simulink model "NormalChopper"  (R2018a)
settings: Solver=VariableStepAuto  StartTime=0.0  StopTime=0.6  RelTol=1e-3  AbsTol=1e-3  EnableMultiTasking=on
values from neighbouring files (symbols this model uses):
  C1 = 200e-6    (= 0.0002)    [test_TFCheck.m]
  C1_ESL = 1e-9    (= 1e-09)    [test_TFCheck.m]
  C1_ESR = 1e-3    (= 0.001)    [test_TFCheck.m]
  C2 = 1000e-6    (= 0.001)    [test_TFCheck.m]
  C2_ESL = 1e-9    (= 1e-09)    [test_TFCheck.m]
  C2_ESR = 1e-3    (= 0.001)    [test_TFCheck.m]
  C_smooth = 400e-6    (= 0.0004)    [test_TFCheck.m]
  current_source = 5.0    (= 5)    [test_TFCheck.m]
  L1 = 1e-6    (= 1e-06)    [test_TFCheck.m]
  L1_R = 1e-3    (= 0.001)    [test_TFCheck.m]
  L2 = 1e-6    (= 1e-06)    [test_TFCheck.m]
  L2_R = 1e-3    (= 0.001)    [test_TFCheck.m]
  L_cable = 10e-6    (= 1e-05)    [test_TFCheck.m]
  L_reactor = 200e-6    (= 0.0002)    [test_TFCheck.m]
  R_cable = 12e-3    (= 0.012)    [test_TFCheck.m]
  R_reactor = 30e-3    (= 0.03)    [test_TFCheck.m]
  sample_time = 1e-6    (= 1e-06)    [test_TFCheck.m]
  SW_duty = 0.5    [ChopperRmsSIm.m]    (also in test_TFCheck.m)
  Vdc = 50    [test_TFCheck.m]
libraries: powerlib x22, powerlib_meascontrol x1
settings Model: Creator=snow_  LastModifiedBy=snow_
settings SolverCC: AutoScaleAbsTol=off
settings DataIOCC: LimitDataPoints=on  MaxDataPoints=10000
settings OptimizationCC: LifeSpan=inf
settings DebuggingCC: AllowSymbolicDim=off  SFUnexpectedBacktrackingDiag=warning  SFNoUnconditionalDefaultTransitionDiag=warning  SFExecutionAtInitializationDiag=none
settings CodeAppCC: StateflowObjectComments=on
settings GRTTargetCC: TargetLangStandard=C89/C90 (ANSI)  GeneratePreprocessorConditionals=Disable all
settings ConfigComp: CovMetricSettings=dw  CovHtmlReporting=on  CovSaveCumulativeToWorkspaceVar=on  CovSaveSingleToWorkspaceVar=on  CovExternalEMLEnable=off  CovSFcnEnable=off
settings SimscapeCC: SimscapeLogType=all  SimscapeLogDataHistory=10000

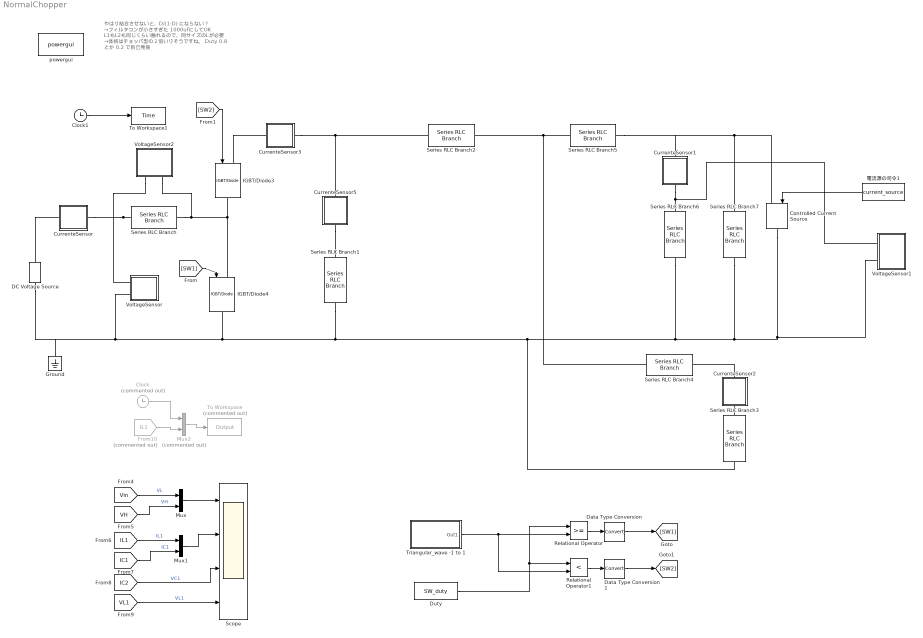
== system NormalChopper ==
  note: やはり結合させないと、D/(1-D)　にならない？
      | →フィルタコンが小さすぎた　1000uFにしてOK
      |
      | L1もL2も同じくらい触れるので、同サイズのLが必要
      | →体格はチョッパ型の２倍いりそうですね。
      |
      | Duty 0.8 とか　0.2 で自己発振
  Clock : Clock  Commented=on
  Clock1 : Clock
  Controlled Current Source : powerlib/Electrical Sources/Controlled Current Source  Initialize=on  Source_Type=AC  Amplitude=0  Phase=0  Frequency=0  Measurements=None
  CurrenteSensor : Subsystem  mask{VariableName=IL1, SampleTime=sample_time}
      mask prompts: VariableName "Simulink:blkprm_prompts:ToWksVarName"
      settings: AttributesFormatString=%<VariableName>
      mask TypeOptions VariableName: To Workspace1/VariableName | Goto/GotoTag
      mask DialogControl VariableName Prompt: 変数名:
      mask Display:
      | disp("Current \n Sensor")
      | port_label('lconn', 1, '+')
      | port_label('rconn', 1, '-')
      | 
      | 
      | %set_param([gcb '/Goto'],'GotoTag',VariableName) % これは使えないっぽい
  CurrenteSensor1 : Subsystem  mask{VariableName=IC2, SampleTime=sample_time}
      mask prompts: VariableName "Simulink:blkprm_prompts:ToWksVarName"
      settings: AttributesFormatString=%<VariableName>
      mask TypeOptions VariableName: To Workspace1/VariableName | Goto/GotoTag
      mask DialogControl VariableName Prompt: 変数名:
      mask Display:
      | disp("Current \n Sensor")
      | port_label('lconn', 1, '+')
      | port_label('rconn', 1, '-')
      | 
      | 
      | %set_param([gcb '/Goto'],'GotoTag',VariableName) % これは使えないっぽい
  CurrenteSensor2 : Subsystem  mask{VariableName=IC3, SampleTime=sample_time}
      mask prompts: VariableName "Simulink:blkprm_prompts:ToWksVarName"
      settings: AttributesFormatString=%<VariableName>
      mask TypeOptions VariableName: To Workspace1/VariableName | Goto/GotoTag
      mask DialogControl VariableName Prompt: 変数名:
      mask Display:
      | disp("Current \n Sensor")
      | port_label('lconn', 1, '+')
      | port_label('rconn', 1, '-')
      | 
      | 
      | %set_param([gcb '/Goto'],'GotoTag',VariableName) % これは使えないっぽい
  CurrenteSensor3 : Subsystem  mask{VariableName=Iin, SampleTime=sample_time}
      mask prompts: VariableName "Simulink:blkprm_prompts:ToWksVarName"
      settings: AttributesFormatString=%<VariableName>
      mask TypeOptions VariableName: To Workspace1/VariableName | Goto/GotoTag
      mask DialogControl VariableName Prompt: 変数名:
      mask Display:
      | % disp("Current \n Sensor")
      | port_label('lconn', 1, '+')
      | port_label('rconn', 1, '-')
      | 
      | 
      | plot(-50,-35,50,50-15,...
      |     [0,9,18,24,29,30,29,24,18,9,0,-9,-18,-24,-29,-30,-29,-24,-18,-9,0],...
      |     0.8*[30,29,24,18,9,0,-9,-18,-24,-29,-30,-29,-24,-18,-9,0,9,18,24,29,30],...
      |     [-15,0,15],0.8*[-15,25,-15],...
      |     [-7,0,7],0.8*[5,5,5]);
  CurrenteSensor5 : Subsystem  mask{VariableName=IC1, SampleTime=sample_time}
      mask prompts: VariableName "Simulink:blkprm_prompts:ToWksVarName"
      settings: AttributesFormatString=%<VariableName>
      mask TypeOptions VariableName: To Workspace1/VariableName | Goto/GotoTag
      mask DialogControl VariableName Prompt: 変数名:
      mask Display:
      | disp("Current \n Sensor")
      | port_label('lconn', 1, '+')
      | port_label('rconn', 1, '-')
      | 
      | 
      | %set_param([gcb '/Goto'],'GotoTag',VariableName) % これは使えないっぽい
  DC Voltage Source : powerlib/Electrical Sources/DC Voltage Source  Amplitude=Vdc  Measurements=None
      settings: AttributesFormatString=DC = %<Amplitude> V
  Data Type Conversion : DataTypeConversion
  Data Type Conversion1 : DataTypeConversion
  "Duty " : Constant  Value=SW_duty
  From10 : From  Commented=on  GotoTag=IL1
  Ground : powerlib/Elements/Ground  LConnTagsString=a
  IGBT/Diode3 : powerlib/Power Electronics/IGBT//Diode  Ron=1e-3  Rs=1e5  Cs=inf  Measurements=off
  IGBT/Diode4 : powerlib/Power Electronics/IGBT//Diode  Ron=1e-3  Rs=1e5  Cs=inf  Measurements=off
  Mux : Mux  Inputs=2
  Mux1 : Mux  Inputs=2
  Mux2 : Mux  Commented=on  Inputs=2
  Relational Operator : RelationalOperator  OutDataTypeStr=boolean  RndMeth=Simplest
  Relational Operator1 : RelationalOperator  Operator=<  OutDataTypeStr=boolean  RndMeth=Simplest
  Scope : Scope  NumInputPorts=4
  Series RLC Branch : powerlib/Elements/Series RLC Branch  LConnTagsString=__new0  RConnTagsString=__new0  BranchType=RL  Resistance=R_reactor  Inductance=L_reactor  SetiL0=off  InitialCurrent=0  Capacitance=1e-6  Setx0=off  InitialVoltage=0  Measurements=None
      settings: AttributesFormatString=|
      | L=%<Inductance> H
      | R=%<Resistance> Ohm
  Series RLC Branch1 : powerlib/Elements/Series RLC Branch  LConnTagsString=__new0  RConnTagsString=__new0  BranchType=C  Resistance=24e-3  Inductance=1000e-6  SetiL0=off  InitialCurrent=0  Capacitance=C_smooth  Setx0=off  InitialVoltage=0  Measurements=None
      settings: AttributesFormatString="C= %<Capacitance>  F"
  Series RLC Branch2 : powerlib/Elements/Series RLC Branch  LConnTagsString=__new0  RConnTagsString=__new0  BranchType=RL  Resistance=R_cable  Inductance=L_cable  SetiL0=off  InitialCurrent=0  Capacitance=1e-6  Setx0=off  InitialVoltage=0  Measurements=None
      settings: AttributesFormatString=|
      | L=%<Inductance> H
      | R=%<Resistance> Ohm
  Series RLC Branch3 : powerlib/Elements/Series RLC Branch  LConnTagsString=__new0  RConnTagsString=__new0  BranchType=RLC  Resistance=C1_ESR  Inductance=C1_ESL  SetiL0=off  InitialCurrent=0  Capacitance=C1  Setx0=off  InitialVoltage=0  Measurements=None
      settings: AttributesFormatString=|
      | L=%<Inductance> H
      | R=%<Resistance> Ohm
  Series RLC Branch4 : powerlib/Elements/Series RLC Branch  LConnTagsString=__new0  RConnTagsString=__new0  BranchType=RL  Resistance=L1_R  Inductance=L1  SetiL0=off  InitialCurrent=0  Capacitance=1e-6  Setx0=off  InitialVoltage=0  Measurements=None
      settings: AttributesFormatString=|
      | L=%<Inductance> H
      | R=%<Resistance> Ohm
  Series RLC Branch5 : powerlib/Elements/Series RLC Branch  LConnTagsString=__new0  RConnTagsString=__new0  BranchType=RL  Resistance=L2_R  Inductance=L2  SetiL0=off  InitialCurrent=0  Capacitance=1e-6  Setx0=off  InitialVoltage=0  Measurements=None
      settings: AttributesFormatString=|
      | L=%<Inductance> H
      | R=%<Resistance> Ohm
  Series RLC Branch6 : powerlib/Elements/Series RLC Branch  LConnTagsString=__new0  RConnTagsString=__new0  BranchType=RLC  Resistance=C2_ESR  Inductance=C2_ESL  SetiL0=off  InitialCurrent=0  Capacitance=C2  Setx0=off  InitialVoltage=0  Measurements=None
      settings: AttributesFormatString=|
      | L=%<Inductance> H
      | R=%<Resistance> Ohm
  Series RLC Branch7 : powerlib/Elements/Series RLC Branch  LConnTagsString=__new0  RConnTagsString=__new0  BranchType=R  Resistance=10e3  Inductance=C2_ESL  SetiL0=off  InitialCurrent=0  Capacitance=C2  Setx0=off  InitialVoltage=0  Measurements=None
      settings: AttributesFormatString=R=%<Resistance> Ohm
  To Workspace : ToWorkspace  Commented=on  VariableName=Output  SampleTime=sample_time
  To Workspace1 : ToWorkspace  VariableName=Time  SampleTime=sample_time
  Triangular_wave -1 to 1 : Subsystem
  VoltageSensor : Subsystem  mask{VariableName=Vin, SampleTime=sample_time}
      mask prompts: VariableName "Simulink:blkprm_prompts:ToWksVarName"
      settings: AttributesFormatString=%<VariableName>
      mask TypeOptions VariableName: To Workspace1/VariableName | Goto/GotoTag
      mask DialogControl VariableName Prompt: 変数名:
      mask Display:
      | %disp("Voltage \n Sensor")
      | port_label('lconn', 1, '+')
      | port_label('lconn', 2, '-')
      | 
      | plot(-50,-35,50,50-15,...
      |     [0,9,18,24,29,30,29,24,18,9,0,-9,-18,-24,-29,-30,-29,-24,-18,-9,0],...
      |     0.8*[30,29,24,18,9,0,-9,-18,-24,-29,-30,-29,-24,-18,-9,0,9,18,24,29,30],...
      |     [-15,0,15],0.8*[15,-20,15]);
  VoltageSensor1 : Subsystem  mask{VariableName=VH, SampleTime=sample_time}
      mask prompts: VariableName "Simulink:blkprm_prompts:ToWksVarName"
      settings: AttributesFormatString=%<VariableName>
      mask TypeOptions VariableName: To Workspace1/VariableName | Goto/GotoTag
      mask DialogControl VariableName Prompt: 変数名:
      mask Display:
      | disp("Voltage \n Sensor")
      | port_label('lconn', 1, '+')
      | port_label('lconn', 2, '-')
      | 
      | 
      | %set_param([gcb '/Goto'],'GotoTag',VariableName) % これは使えないっぽい
  VoltageSensor2 : Subsystem  mask{VariableName=VL1, SampleTime=sample_time}
      mask prompts: VariableName "Simulink:blkprm_prompts:ToWksVarName"
      settings: AttributesFormatString=%<VariableName>
      mask TypeOptions VariableName: To Workspace1/VariableName | Goto/GotoTag
      mask DialogControl VariableName Prompt: 変数名:
      mask Display:
      | disp("Voltage \n Sensor")
      | port_label('lconn', 1, '+')
      | port_label('lconn', 2, '-')
      | 
      | 
      | %set_param([gcb '/Goto'],'GotoTag',VariableName) % これは使えないっぽい
  powergui : powerlib/powergui  Priority=1  SimulationMode=Continuous  SampleTime=50e-6  frequency=60  Iterations=50  frequencyindice=0  Pbase=100e6  ErrMax=1e-4  UnitsV=kV  UnitsW=MW  buscounter=0  FunctionMessages=off  echomessages=off  EnableUseOfTLC=off  CurrentSourceSwitches=off  DisableSnubberDevices=off  DisableRonSwitches=off  DisableVfSwitches=off  DisplayEquations=off  SolverType=Tustin/Backward Euler (TBE)  Interpol=off  ExternalGateDelay=off  methode=off  Ts=100  x0status=blocks  SPID=on  SwTol=0  HookPort=off  RestoreLinks=warning  ResistiveCurrentMeasurement=off  Frange=[0:2:500]  Ylog=off  Xlog=on  ShowGrid=off  save=off  variable=ZData  structure=0  ZoomFFT=off  StartTime=0.0  cycles=1  DisplayStyle=1  fundamental=60  FreqAxis=off  MaxFrequency=1000  frequencyindicesteady=1  RmsSteady=1  display=off
  電流源の司令1 : Constant  Value=current_source
  wires:
  Relational Operator/1 -> Data Type Conversion/1
  Relational Operator1/1 -> Data Type Conversion1/1
  [SW1] -> IGBT/Diode4/1
  Mux/1 -> Scope/1
  Data Type Conversion1/1 -> [SW2]
  Data Type Conversion/1 -> [SW1]
  [Vin] -> Mux/1  "VL"
  [VH] -> Mux/2  "VH"
  [IL1] -> Mux1/1  "IL1"
  [IC1] -> Mux1/2  "IC1"
  Mux1/1 -> Scope/2
  [IC2] -> Scope/3  "VC1"
  [VL1] -> Scope/4  "VL1"
  [SW2] -> IGBT/Diode3/1
  "Duty "/1 -> Relational Operator1/1, Relational Operator/1
  From10/1 -> Mux2/2
  Clock/1 -> Mux2/1
  Mux2/1 -> To Workspace/1
  Triangular_wave -1 to 1/1(Out1) -> Relational Operator1/2, Relational Operator/2
  電流源の司令1/1 -> Controlled Current Source/1
  Clock1/1 -> To Workspace1/1
  connections:
  Series RLC Branch4/LConn1 -- Series RLC Branch5/LConn1 -- Series RLC Branch2/RConn1
  Controlled Current Source/RConn1 -- VoltageSensor1/LConn2 -- Series RLC Branch7/RConn1 -- Series RLC Branch6/RConn1 -- Series RLC Branch3/RConn1 -- Series RLC Branch1/RConn1 -- VoltageSensor/LConn2 -- Ground/LConn1 -- DC Voltage Source/LConn1 -- IGBT/Diode4/RConn1
  Series RLC Branch/RConn1 -- VoltageSensor2/LConn2 -- IGBT/Diode3/RConn1 -- IGBT/Diode4/LConn1
  CurrenteSensor/LConn1 -- DC Voltage Source/RConn1
  Series RLC Branch/LConn1 -- VoltageSensor2/LConn1 -- CurrenteSensor/RConn1 -- VoltageSensor/LConn1
  CurrenteSensor2/RConn1 -- Series RLC Branch3/LConn1
  CurrenteSensor1/RConn1 -- VoltageSensor1/LConn1 -- Series RLC Branch6/LConn1
  Series RLC Branch2/LConn1 -- CurrenteSensor5/LConn1 -- CurrenteSensor3/RConn1
  CurrenteSensor5/RConn1 -- Series RLC Branch1/LConn1
  Series RLC Branch7/LConn1 -- Controlled Current Source/LConn1 -- CurrenteSensor1/LConn1 -- Series RLC Branch5/RConn1
  CurrenteSensor2/LConn1 -- Series RLC Branch4/RConn1
  CurrenteSensor3/LConn1 -- IGBT/Diode3/LConn1

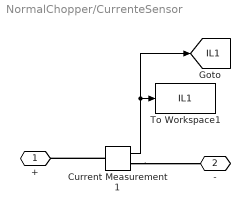
== system NormalChopper/CurrenteSensor ==
  Current Measurement1 : powerlib/Measurements/Current Measurement  PhasorSimulation=off  OutputType=Complex  PSBequivalent=0
  To Workspace1 : ToWorkspace  VariableName=IL1  SampleTime=sample_time
  + : PMIOPort  Side=Left
  - : PMIOPort  Port=2  Side=Right
  tag scope: IL1=global
  wires:
  Current Measurement1/1 -> [IL1], To Workspace1/1
  connections:
  Current Measurement1/LConn1 -- +/RConn1
  Current Measurement1/RConn1 -- -/RConn1

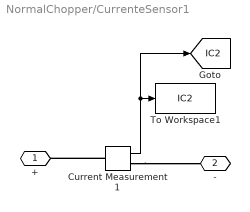
== system NormalChopper/CurrenteSensor1 ==
  Current Measurement1 : powerlib/Measurements/Current Measurement  PhasorSimulation=off  OutputType=Complex  PSBequivalent=0
  To Workspace1 : ToWorkspace  VariableName=IC2  SampleTime=sample_time
  + : PMIOPort  Side=Left
  - : PMIOPort  Port=2  Side=Right
  tag scope: IC2=global
  wires:
  Current Measurement1/1 -> [IC2], To Workspace1/1
  connections:
  Current Measurement1/LConn1 -- +/RConn1
  Current Measurement1/RConn1 -- -/RConn1

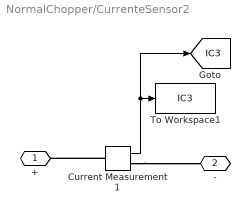
== system NormalChopper/CurrenteSensor2 ==
  Current Measurement1 : powerlib/Measurements/Current Measurement  PhasorSimulation=off  OutputType=Complex  PSBequivalent=0
  To Workspace1 : ToWorkspace  VariableName=IC3  SampleTime=sample_time
  + : PMIOPort  Side=Left
  - : PMIOPort  Port=2  Side=Right
  tag scope: IC3=global
  wires:
  Current Measurement1/1 -> [IC3], To Workspace1/1
  connections:
  Current Measurement1/LConn1 -- +/RConn1
  Current Measurement1/RConn1 -- -/RConn1

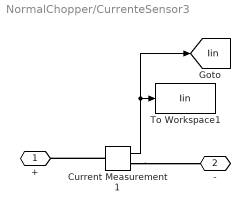
== system NormalChopper/CurrenteSensor3 ==
  Current Measurement1 : powerlib/Measurements/Current Measurement  PhasorSimulation=off  OutputType=Complex  PSBequivalent=0
  To Workspace1 : ToWorkspace  VariableName=Iin  SampleTime=sample_time
  + : PMIOPort  Side=Left
  - : PMIOPort  Port=2  Side=Right
  tag scope: Iin=global
  wires:
  Current Measurement1/1 -> [Iin], To Workspace1/1
  connections:
  Current Measurement1/LConn1 -- +/RConn1
  Current Measurement1/RConn1 -- -/RConn1

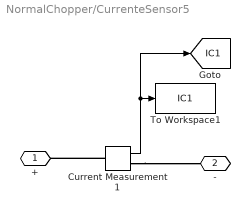
== system NormalChopper/CurrenteSensor5 ==
  Current Measurement1 : powerlib/Measurements/Current Measurement  PhasorSimulation=off  OutputType=Complex  PSBequivalent=0
  To Workspace1 : ToWorkspace  VariableName=IC1  SampleTime=sample_time
  + : PMIOPort  Side=Left
  - : PMIOPort  Port=2  Side=Right
  tag scope: IC1=global
  wires:
  Current Measurement1/1 -> [IC1], To Workspace1/1
  connections:
  Current Measurement1/LConn1 -- +/RConn1
  Current Measurement1/RConn1 -- -/RConn1

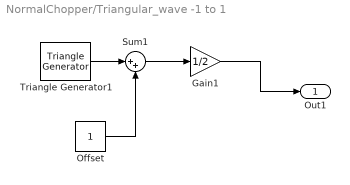
== system NormalChopper/Triangular_wave -1 to 1 ==
  Gain1 : Gain  Gain=1/2
  "Offset " : Constant
  Sum1 : Sum  Inputs=|++
  Triangle Generator1 : powerlib_meascontrol/Pulse & Signal Generators/Triangle Generator  Freq=FSW  Phase=0  Ts=0
      settings: AttributesFormatString=Freq = %<Freq> Hz
  Out1 : Outport
  wires:
  "Offset "/1 -> Sum1/2
  Sum1/1 -> Gain1/1
  Triangle Generator1/1 -> Sum1/1
  Gain1/1 -> Out1/1

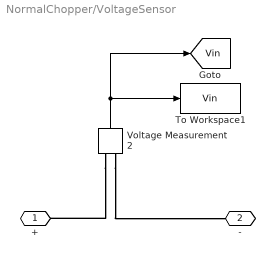
== system NormalChopper/VoltageSensor ==
  To Workspace1 : ToWorkspace  VariableName=Vin  SampleTime=SampleTime
  Voltage Measurement2 : powerlib/Measurements/Voltage Measurement  PhasorSimulation=off  OutputType=Complex  PSBequivalent=0
  + : PMIOPort  Side=Left
  - : PMIOPort  Port=2  Side=Left
  tag scope: Vin=global
  wires:
  Voltage Measurement2/1 -> [Vin], To Workspace1/1
  connections:
  Voltage Measurement2/LConn1 -- +/RConn1
  Voltage Measurement2/LConn2 -- -/RConn1

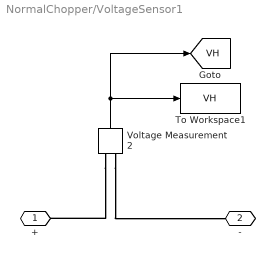
== system NormalChopper/VoltageSensor1 ==
  To Workspace1 : ToWorkspace  VariableName=VH  SampleTime=SampleTime
  Voltage Measurement2 : powerlib/Measurements/Voltage Measurement  PhasorSimulation=off  OutputType=Complex  PSBequivalent=0
  + : PMIOPort  Side=Left
  - : PMIOPort  Port=2  Side=Left
  tag scope: VH=global
  wires:
  Voltage Measurement2/1 -> [VH], To Workspace1/1
  connections:
  Voltage Measurement2/LConn1 -- +/RConn1
  Voltage Measurement2/LConn2 -- -/RConn1

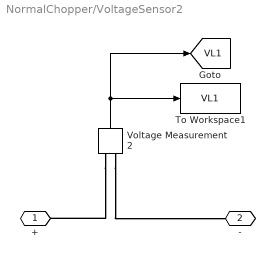
== system NormalChopper/VoltageSensor2 ==
  To Workspace1 : ToWorkspace  VariableName=VL1  SampleTime=SampleTime
  Voltage Measurement2 : powerlib/Measurements/Voltage Measurement  PhasorSimulation=off  OutputType=Complex  PSBequivalent=0
  + : PMIOPort  Side=Left
  - : PMIOPort  Port=2  Side=Left
  tag scope: VL1=global
  wires:
  Voltage Measurement2/1 -> [VL1], To Workspace1/1
  connections:
  Voltage Measurement2/LConn1 -- +/RConn1
  Voltage Measurement2/LConn2 -- -/RConn1
